simulink model "ELEC522_PROJECT2"  (Simulink 8.9)
settings: Solver=VariableStepAuto  StartTime=0.0  StopTime=10  RelTol=1e-3
undefined symbols (not defined in the file): A, N
libraries: xbsIndex_r4 x127, JTAGRuntimeCosim_r4 x1
(part 1 of 2)
settings Model: Creator=Kenny_LR  LastModifiedBy=rl59
settings DataIOCC: LimitDataPoints=off  SaveFormat=Dataset  SignalLoggingSaveFormat=Dataset
settings OptimizationCC: LifeSpan=auto
settings DebuggingCC: UnderspecifiedInitializationDetection=Simplified  MergeDetectMultiDrivingBlocksExec=error  FcnCallInpInsideContextMsg=error  StateNameClashWarn=none  SFUnexpectedBacktrackingDiag=error  SFNoUnconditionalDefaultTransitionDiag=error  SFExecutionAtInitializationDiag=warning
settings HardwareCC: ProdBitPerPointer=64  ProdBitPerSizeT=64  ProdBitPerPtrDiffT=64  ProdLargestAtomicFloat=Float  ProdIntDivRoundTo=Zero  ProdEndianess=LittleEndian  ProdWordSize=64  ProdHWDeviceType=Intel->x86-64 (Windows64)
settings ModelReferenceCC: PropagateSignalLabelsOutOfModel=on
settings GRTTargetCC: TargetLangStandard=C99 (ISO)  GeneratePreprocessorConditionals=Use local settings  CombineOutputUpdateFcns=on  GRTInterface=off
settings ConfigComp: CovMetricSettings=dwe  CovHtmlReporting=off  CovSaveCumulativeToWorkspaceVar=off  CovSaveSingleToWorkspaceVar=off  CovExternalEMLEnable=on

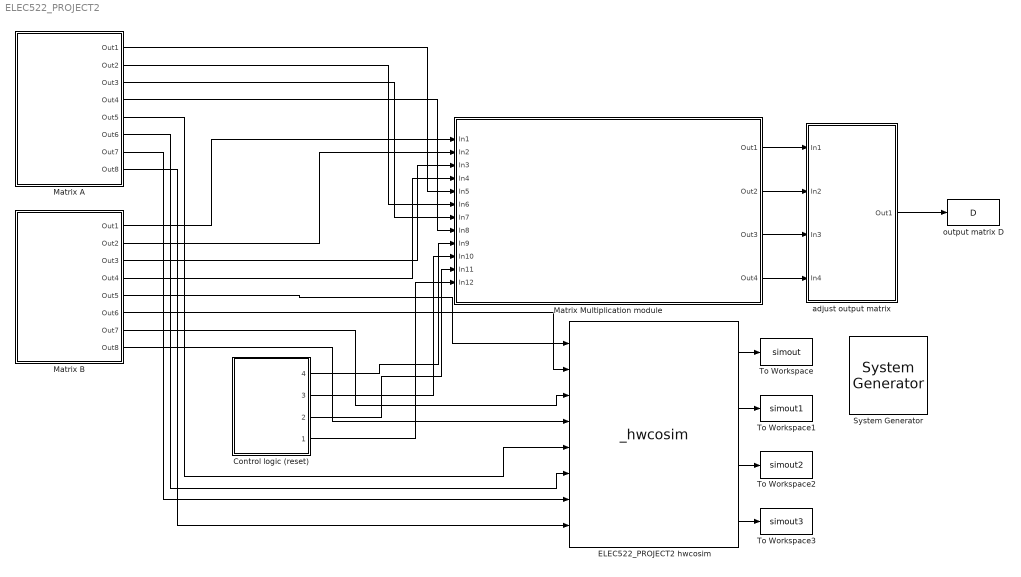
== system ELEC522_PROJECT2 ==
  " System Generator" : xbsIndex_r4/ System Generator  Tag=genX  xilinxfamily=zynq  part=xc7z020  speed=-1  package=clg484  synthesis_tool=Vivado  clock_wrapper=Clock Enables  directory=./netlist  proj_type=Vivado  Synth_file=Vivado Synthesis Defaults  Impl_file=Vivado Implementation Defaults  testbench=off  simulink_period=1  sysclk_period=10  dcm_input_clock_period=10  incr_netlist=off  trim_vbits=Everywhere in SubSystem  dbl_ovrd=According to Block Masks  core_generation=According to Block Masks  run_coregen=off  deprecated_control=off  eval_field=0  block_type=sysgen
  Control logic (reset) : Subsystem
  ELEC522_PROJECT2 hwcosim : JTAGRuntimeCosim_r4/_hwcosim  clkSrc=Single Stepped  hasCombinationalPath=on  bitfileName=C:\Users\rl59\Desktop\netlist\elec522_project2.bit  skipConfig=off  dispPartInfo=off  useZynqReconfigScript=on  cable=Auto Detect  speed=N/A  cablePort=N/A  cableLocation=Local  shareCable=off  design_xtable=|  engineDll=JTAGCosimEngine.dll  cableWaitTime=10  bscanPos=-1  IRLengths=[]  useWaitBox=1  hasBufgmux=on  Scheme=Cosim  useCmdProc=1  hasProc=0  useImpact=0  printLogFile=0  userChain=2  block_type=jtagcosim
      | {
      |     'clkWrapper' => 'elec522_project2',
      |     'burstMode' => false,
      |     'burstFifoDepth' => '1024',
      |     'shared_memories' => {},
      |     'clocksGcd' => 1,
      |     'device' => {
      |       'family' => 'zynq',
      |       'part' => 'xc7z020',
      |       'package' => 'clg484',
      |       'speed' => '-1',
      |     },
      |     'ports' => {
      |       'gateway_in3' => {
      |         'direction' => 'in',
      |         'width' => 16,
      |         'name' => 'gateway_in3',
      |         'period' => 1,
      |         'icon_text' => 'Gateway In3',
      |         'type' => 'UFix_16_0',
      |         'arithmetic_type' => 'xlUnsigned',
      |         'dat_file' => 'elec522_project2_matrix_b_gateway_in3.dat',
      |         'bin_pt' => 0,
      |         'addr_offset' => 0,
      |         'bd_port_index' => 0,
      |       },
      |       'gateway_in2' => {
      |         'direction' => 'in',
      |         'width' => 16,
      |         'name' => 'gateway_in2',
      |         'period' => 1,
      |         'icon_text' => 'Gateway In2',
      |         'type' => 'UFix_16_0',
      |         'arithmetic_type' => 'xlUnsigned',
      |         'dat_file' => 'elec522_project2_matrix_b_gateway_in2.dat',
      |         'bin_pt' => 0,
      |         'addr_offset' => 4,
      |         'bd_port_index' => 1,
      |       },
      |       'gateway_in1' => {
      |         'direction' => 'in',
      |         'width' => 16,
      |         'name' => 'gateway_in1',
      |         'period' => 1,
      |         'icon_text' => 'Gateway In1',
      |         'type' => 'UFix_16_0',
      |         'arithmetic_type' => 'xlUnsigned',
      |         'dat_file' => 'elec522_project2_matrix_b_gateway_in1.dat',
      |         'bin_pt' => 0,
      |         'addr_offset' => 8,
      |         'bd_port_index' => 2,
      |       },
      |       'gateway_in' => {
      |         'direction' => 'in',
      |         'width' => 16,
      |         'name' => 'gateway_in',
      |         'period' => 1,
      |         'icon_text' => 'Gateway In',
      |         'type' => 'UFix_16_0',
      |         'arithmetic_type' => 'xlUnsigned',
      |         'dat_file' => 'elec522_project2_matrix_b_gateway_in.dat',
      |         'bin_pt' => 0,
      |         'addr_offset' => 12,
      |         'bd_port_index' => 3,
      |       },
      |       'gateway_in7' => {
      |         'direction' => 'in',
      |         'width' => 16,
      |         'name' => 'gateway_in7',
      |         'period' => 1,
      |         'icon_text' => 'Gateway In7',
      |         'type' => 'UFix_16_0',
      |         'arithmetic_type' => 'xlUnsigned',
      |         'dat_file' => 'elec522_project2_matrix_a_gateway_in7.dat',
      |         'bin_pt' => 0,
      |         'addr_offset' => 16,
      |         'bd_port_index' => 4,
      |       },
      |       'gateway_in6' => {
      |         'direction' => 'in',
      |         'width' => 16,
      |         'name' => 'gateway_in6',
      |         'period' => 1,
      |         'icon_text' => 'Gateway In6',
      |         'type' => 'UFix_16_0',
      |         'arithmetic_type' => 'xlUnsigned',
      |         'dat_file' => 'elec522_project2_matrix_a_gateway_in6.dat',
      |         'bin_pt' => 0,
      |         'addr_offset' => 20,
      |         'bd_port_index' => 5,
      |       },
      |       'gateway_in5' => {
      |         'direction' => 'in',
      |         'width' => 16,
      |         'name' => 'gateway_in5',
      |         'period' => 1,
      |         'icon_text' => 'Gateway In5',
      |         'type' => 'UFix_16_0',
      |         'arithmetic_type' => 'xlUnsigned',
      |         'dat_file' => 'elec522_project2_matrix_a_gateway_in5.dat',
      |         'bin_pt' => 0,
      |         'addr_offset' => 24,
      |         'bd_port_index' => 6,
      |       },
      |       'gateway_in4' => {
      |         'direction' => 'in',
      |         'width' => 16,
      |         'name' => 'gateway_in4',
      |         'period' => 1,
      |         'icon_text' => 'Gateway In4',
      |         'type' => 'UFix_16_0',
      |         'arithmetic_type' => 'xlUnsigned',
      |         'dat_file' => 'elec522_project2_matrix_a_gateway_in4.dat',
      |         'bin_pt' => 0,
      |         'addr_offset' => 28,
      |         'bd_port_index' => 7,
      |       },
      |       'gateway_out' => {
      |         'direction' => 'out',
      |         'width' => 28,
      |         'name' => 'gateway_out',
      |         'period' => 1,
      |         'icon_text' => 'Gateway Out',
      |         'type' => 'UFix_28_0',
      |         'arithmetic_type' => 'xlUnsigned',
      |         'dat_file' => 'elec522_project2_adjust_output_matrix_gateway_out.dat',
      |         'bin_pt' => 0,
      |         'addr_offset' => 32,
      |         'bd_port_index' => 0,
      |       },
      |       'gateway_out1' => {
      |         'direction' => 'out',
      |         'width' => 28,
      |         'name' => 'gateway_out1',
      |         'period' => 1,
      |         'icon_text' => 'Gateway Out1',
      |         'type' => 'UFix_28_0',
      |         'arithmetic_type' => 'xlUnsigned',
      |         'dat_file' => 'elec522_project2_adjust_output_matrix_gateway_out1.dat',
      |         'bin_pt' => 0,
      |         'addr_offset' => 36,
      |         'bd_port_index' => 1,
      |       },
      |       'gateway_out2' => {
      |         'direction' => 'out',
      |         'width' => 28,
      |         'name' => 'gateway_out2',
      |         'period' => 1,
      |         'icon_text' => 'Gateway Out2',
      |         'type' => 'UFix_28_0',
      |         'arithmetic_type' => 'xlUnsigned',
      |         'dat_file' => 'elec522_project2_adjust_output_matrix_gateway_out2.dat',
      |         'bin_pt' => 0,
      |         'addr_offset' => 40,
      |         'bd_port_index' => 2,
      |       },
      |       'gateway_out3' => {
      |         'direction' => 'out',
      |         'width' => 28,
      |         'name' => 'gateway_out3',
      |         'period' => 1,
      |         'icon_text' => 'Gateway Out3',
      |         'type' => 'UFix_28_0',
      |         'arithmetic_type' => 'xlUnsigned',
      |         'dat_file' => 'elec522_project2_adjust_output_matrix_gateway_out3.dat',
      |         'bin_pt' => 0,
      |         'addr_offset' => 44,
      |         'bd_port_index' => 3,
      |       },
      |     },
      |   }
  Matrix A : Subsystem
  Matrix B : Subsystem
  Matrix Multiplication module : Subsystem
  To Workspace : ToWorkspace  VariableName=simout  SaveFormat=Timeseries  SampleTime=-1
  To Workspace1 : ToWorkspace  VariableName=simout1  SaveFormat=Timeseries  SampleTime=-1
  To Workspace2 : ToWorkspace  VariableName=simout2  SaveFormat=Timeseries  SampleTime=-1
  To Workspace3 : ToWorkspace  VariableName=simout3  SaveFormat=Timeseries  SampleTime=-1
  "adjust output matrix " : Subsystem
  output matrix D : ToWorkspace  VariableName=D  SampleTime=1
      settings: MaxDataPoints=4
  wires:
  Control logic (reset)/1(4) -> Matrix Multiplication module/9(In9)
  Control logic (reset)/2(3) -> Matrix Multiplication module/10(In10)
  Control logic (reset)/3(2) -> Matrix Multiplication module/11(In11)
  Control logic (reset)/4(1) -> Matrix Multiplication module/12(In12)
  ELEC522_PROJECT2 hwcosim/1 -> To Workspace/1
  ELEC522_PROJECT2 hwcosim/2 -> To Workspace1/1
  ELEC522_PROJECT2 hwcosim/3 -> To Workspace2/1
  ELEC522_PROJECT2 hwcosim/4 -> To Workspace3/1
  Matrix A/1(Out1) -> Matrix Multiplication module/5(In5)
  Matrix A/2(Out2) -> Matrix Multiplication module/6(In6)
  Matrix A/3(Out3) -> Matrix Multiplication module/7(In7)
  Matrix A/4(Out4) -> Matrix Multiplication module/8(In8)
  Matrix A/5(Out5) -> ELEC522_PROJECT2 hwcosim/5
  Matrix A/6(Out6) -> ELEC522_PROJECT2 hwcosim/6
  Matrix A/7(Out7) -> ELEC522_PROJECT2 hwcosim/7
  Matrix A/8(Out8) -> ELEC522_PROJECT2 hwcosim/8
  Matrix B/1(Out1) -> Matrix Multiplication module/1(In1)
  Matrix B/2(Out2) -> Matrix Multiplication module/2(In2)
  Matrix B/3(Out3) -> Matrix Multiplication module/3(In3)
  Matrix B/4(Out4) -> Matrix Multiplication module/4(In4)
  Matrix B/5(Out5) -> ELEC522_PROJECT2 hwcosim/1
  Matrix B/6(Out6) -> ELEC522_PROJECT2 hwcosim/2
  Matrix B/7(Out7) -> ELEC522_PROJECT2 hwcosim/3
  Matrix B/8(Out8) -> ELEC522_PROJECT2 hwcosim/4
  Matrix Multiplication module/1(Out1) -> "adjust output matrix "/1(In1)
  Matrix Multiplication module/2(Out2) -> "adjust output matrix "/2(In2)
  Matrix Multiplication module/3(Out3) -> "adjust output matrix "/3(In3)
  Matrix Multiplication module/4(Out4) -> "adjust output matrix "/4(In4)
  "adjust output matrix "/1(Out1) -> output matrix D/1

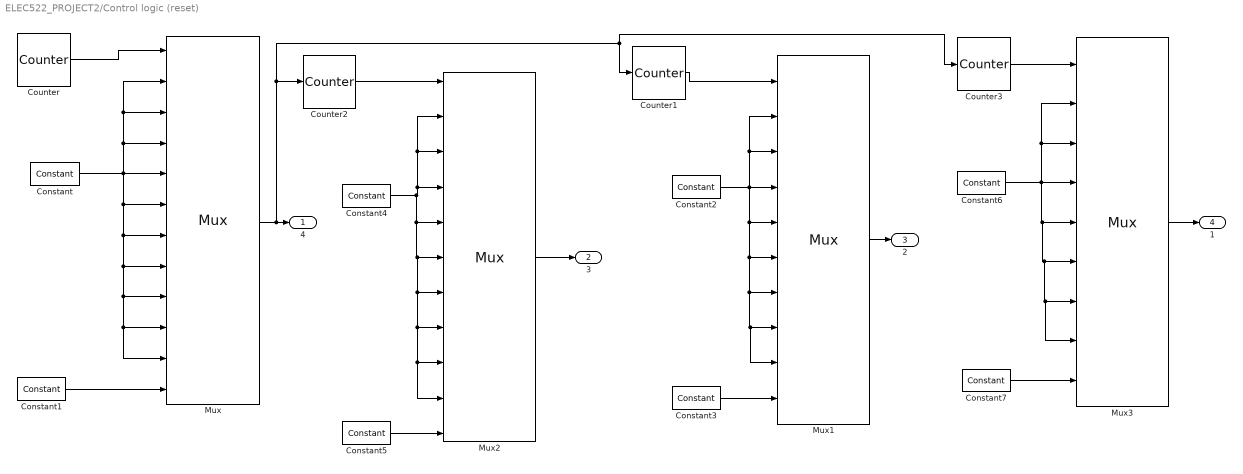
== system ELEC522_PROJECT2/Control logic (reset) ==
  Constant{,2,4,6} (4 alike) : xbsIndex_r4/Constant  const=0  gui_display_data_type=Boolean  arith_type=Boolean  n_bits=1  bin_pt=0  preci_type=Single  exp_width=8  frac_width=24  explicit_period=on  period=1  equ=P=C  opselect=C  inp2=PCIN>>17  opr=+  inp1=P  carry=CIN  dbl_ovrd=off  block_type=constant
  Constant{1,3,5,7} (4 alike) : xbsIndex_r4/Constant  const=1  gui_display_data_type=Boolean  arith_type=Boolean  n_bits=1  bin_pt=0  preci_type=Single  exp_width=8  frac_width=24  explicit_period=on  period=1  equ=P=C  opselect=C  inp2=PCIN>>17  opr=+  inp1=P  carry=CIN  dbl_ovrd=off  block_type=constant
  Counter : xbsIndex_r4/Counter  cnt_type=Count Limited  cnt_to=10  operation=Up  start_count=0  cnt_by_val=1  arith_type=Unsigned  n_bits=4  bin_pt=0  load_pin=off  rst=off  en=off  explicit_period=on  period=1  use_behavioral_HDL=off  implementation=Fabric  dbl_ovrd=off  block_type=counter
  Counter1 : xbsIndex_r4/Counter  cnt_type=Count Limited  cnt_to=8  operation=Up  start_count=0  cnt_by_val=1  arith_type=Unsigned  n_bits=4  bin_pt=0  load_pin=off  rst=on  en=off  explicit_period=on  period=1  use_behavioral_HDL=off  implementation=Fabric  dbl_ovrd=off  block_type=counter
  Counter2 : xbsIndex_r4/Counter  cnt_type=Count Limited  cnt_to=9  operation=Up  start_count=0  cnt_by_val=1  arith_type=Unsigned  n_bits=4  bin_pt=0  load_pin=off  rst=on  en=off  explicit_period=on  period=1  use_behavioral_HDL=off  implementation=Fabric  dbl_ovrd=off  block_type=counter
  Counter3 : xbsIndex_r4/Counter  cnt_type=Count Limited  cnt_to=7  operation=Up  start_count=0  cnt_by_val=1  arith_type=Unsigned  n_bits=3  bin_pt=0  load_pin=off  rst=on  en=off  explicit_period=on  period=1  use_behavioral_HDL=off  implementation=Fabric  dbl_ovrd=off  block_type=counter
  Mux : xbsIndex_r4/Mux  inputs=11  en=off  latency=0  precision=Full  arith_type=Unsigned  n_bits=16  bin_pt=14  quantization=Truncate  overflow=Wrap  dbl_ovrd=off  block_type=mux
  Mux1 : xbsIndex_r4/Mux  inputs=9  en=off  latency=0  precision=Full  arith_type=Unsigned  n_bits=16  bin_pt=14  quantization=Truncate  overflow=Wrap  dbl_ovrd=off  block_type=mux
  Mux2 : xbsIndex_r4/Mux  inputs=10  en=off  latency=0  precision=Full  arith_type=Unsigned  n_bits=16  bin_pt=14  quantization=Truncate  overflow=Wrap  dbl_ovrd=off  block_type=mux
  Mux3 : xbsIndex_r4/Mux  inputs=8  en=off  latency=0  precision=Full  arith_type=Unsigned  n_bits=16  bin_pt=14  quantization=Truncate  overflow=Wrap  dbl_ovrd=off  block_type=mux
  4 : Outport
  3 : Outport  Port=2
  2 : Outport  Port=3
  1 : Outport  Port=4
  wires:
  Mux/1 -> Counter3/1, Counter1/1, Counter2/1, 4/1
  Counter/1 -> Mux/1
  Constant1/1 -> Mux/12
  Counter1/1 -> Mux1/1
  Counter2/1 -> Mux2/1
  Counter3/1 -> Mux3/1
  Constant5/1 -> Mux2/11
  Constant3/1 -> Mux1/10
  Mux2/1 -> 3/1
  Mux1/1 -> 2/1
  Mux3/1 -> 1/1
  Constant7/1 -> Mux3/9
  Constant/1 -> Mux/11, Mux/10, Mux/9, Mux/8, Mux/7, Mux/6, Mux/5, Mux/4, Mux/3, Mux/2
  Constant4/1 -> Mux2/10, Mux2/9, Mux2/8, Mux2/7, Mux2/6, Mux2/5, Mux2/4, Mux2/3, Mux2/2
  Constant2/1 -> Mux1/9, Mux1/8, Mux1/7, Mux1/6, Mux1/5, Mux1/4, Mux1/3, Mux1/2
  Constant6/1 -> Mux3/8, Mux3/7, Mux3/6, Mux3/5, Mux3/4, Mux3/3, Mux3/2

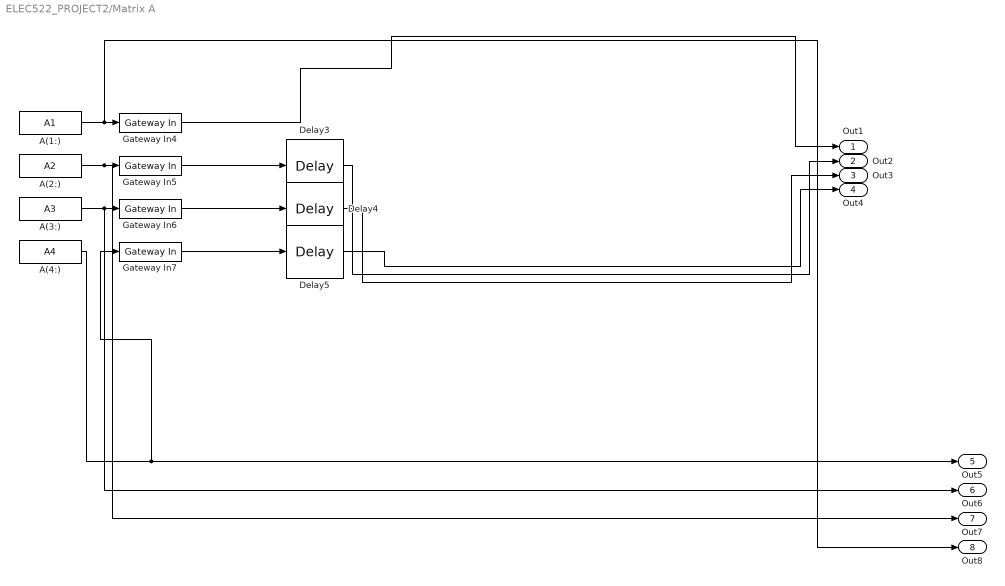
== system ELEC522_PROJECT2/Matrix A ==
  A(1:) : FromWorkspace  VariableName=A1  SampleTime=1  OutputAfterFinalValue=Setting to zero
  A(2:) : FromWorkspace  VariableName=A2  SampleTime=0  OutputAfterFinalValue=Setting to zero
  A(3:) : FromWorkspace  VariableName=A3  SampleTime=0  OutputAfterFinalValue=Setting to zero
  A(4:) : FromWorkspace  VariableName=A4  SampleTime=0  OutputAfterFinalValue=Setting to zero
  Delay3 : xbsIndex_r4/Delay  rst=off  infoeditControl=Selection of Reset will increase slice count due to use of real FFs and instead of SRLs  en=off  latency=1  reg_retiming=off  dbl_ovrd=off  block_type=delay
  Delay4 : xbsIndex_r4/Delay  rst=off  infoeditControl=Selection of Reset will increase slice count due to use of real FFs and instead of SRLs  en=off  latency=2  reg_retiming=off  dbl_ovrd=off  block_type=delay
  Delay5 : xbsIndex_r4/Delay  rst=off  infoeditControl=Selection of Reset will increase slice count due to use of real FFs and instead of SRLs  en=off  latency=3  reg_retiming=off  dbl_ovrd=off  block_type=delay
  Gateway In{4..7} (4 alike) : xbsIndex_r4/Gateway In  gui_display_data_type=Fixed-point  arith_type=Unsigned  n_bits=16  bin_pt=0  preci_type=Single  exp_width=8  frac_width=24  rows=1  columns=1  quantization="Round  (unbiased: +/- Inf)"  overflow=Saturate  period=1  UseAsADC=off  ADCChannel='1'  interface=None  automatic_assignment=on  address_offset=hex2dec('00')  intf_name=''  intf_description=''  default_value=0  timing_constraint=None  locs_specified=off  LOCs={}  io_standard={}  inherit_from_input=off  hdl_port=on  dbl_ovrd=off  block_type=gatewayin
  Out1 : Outport
  Out2 : Outport  Port=2
  Out3 : Outport  Port=3
  Out4 : Outport  Port=4
  Out5 : Outport  Port=5
  Out6 : Outport  Port=6
  Out7 : Outport  Port=7
  Out8 : Outport  Port=8
  wires:
  Gateway In6/1 -> Delay4/1
  A(2:)/1 -> Out7/1, Gateway In5/1
  Gateway In5/1 -> Delay3/1
  Gateway In7/1 -> Delay5/1
  A(1:)/1 -> Out8/1, Gateway In4/1
  A(3:)/1 -> Out6/1, Gateway In6/1
  A(4:)/1 -> Out5/1, Gateway In7/1
  Gateway In4/1 -> Out1/1
  Delay3/1 -> Out2/1
  Delay4/1 -> Out3/1
  Delay5/1 -> Out4/1

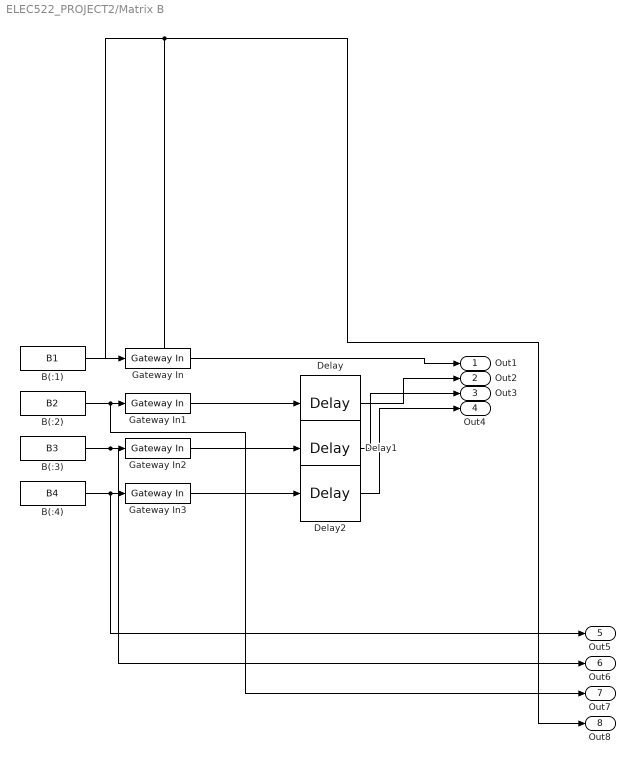
== system ELEC522_PROJECT2/Matrix B ==
  B(:1) : FromWorkspace  VariableName=B1  SampleTime=1  OutputAfterFinalValue=Setting to zero
  B(:2) : FromWorkspace  VariableName=B2  SampleTime=1  OutputAfterFinalValue=Setting to zero
  B(:3) : FromWorkspace  VariableName=B3  SampleTime=1  OutputAfterFinalValue=Setting to zero
  B(:4) : FromWorkspace  VariableName=B4  SampleTime=1  OutputAfterFinalValue=Setting to zero
  Delay : xbsIndex_r4/Delay  rst=off  infoeditControl=Selection of Reset will increase slice count due to use of real FFs and instead of SRLs  en=off  latency=1  reg_retiming=off  dbl_ovrd=off  block_type=delay
  Delay1 : xbsIndex_r4/Delay  rst=off  infoeditControl=Selection of Reset will increase slice count due to use of real FFs and instead of SRLs  en=off  latency=2  reg_retiming=off  dbl_ovrd=off  block_type=delay
  Delay2 : xbsIndex_r4/Delay  rst=off  infoeditControl=Selection of Reset will increase slice count due to use of real FFs and instead of SRLs  en=off  latency=3  reg_retiming=off  dbl_ovrd=off  block_type=delay
  Gateway In{,1..3} (4 alike) : xbsIndex_r4/Gateway In  gui_display_data_type=Fixed-point  arith_type=Unsigned  n_bits=16  bin_pt=0  preci_type=Single  exp_width=8  frac_width=24  rows=1  columns=1  quantization="Round  (unbiased: +/- Inf)"  overflow=Saturate  period=1  UseAsADC=off  ADCChannel='1'  interface=None  automatic_assignment=on  address_offset=hex2dec('00')  intf_name=''  intf_description=''  default_value=0  timing_constraint=None  locs_specified=off  LOCs={}  io_standard={}  inherit_from_input=off  hdl_port=on  dbl_ovrd=off  block_type=gatewayin
  Out1 : Outport
  Out2 : Outport  Port=2
  Out3 : Outport  Port=3
  Out4 : Outport  Port=4
  Out5 : Outport  Port=5
  Out6 : Outport  Port=6
  Out7 : Outport  Port=7
  Out8 : Outport  Port=8
  wires:
  B(:2)/1 -> Out7/1, Gateway In1/1
  B(:1)/1 -> Out8/1, Gateway In/1
  B(:3)/1 -> Out6/1, Gateway In2/1
  Gateway In2/1 -> Delay1/1
  Gateway In3/1 -> Delay2/1
  Gateway In1/1 -> Delay/1
  B(:4)/1 -> Out5/1, Gateway In3/1
  Gateway In/1 -> Out1/1
  Delay/1 -> Out2/1
  Delay1/1 -> Out3/1
  Delay2/1 -> Out4/1

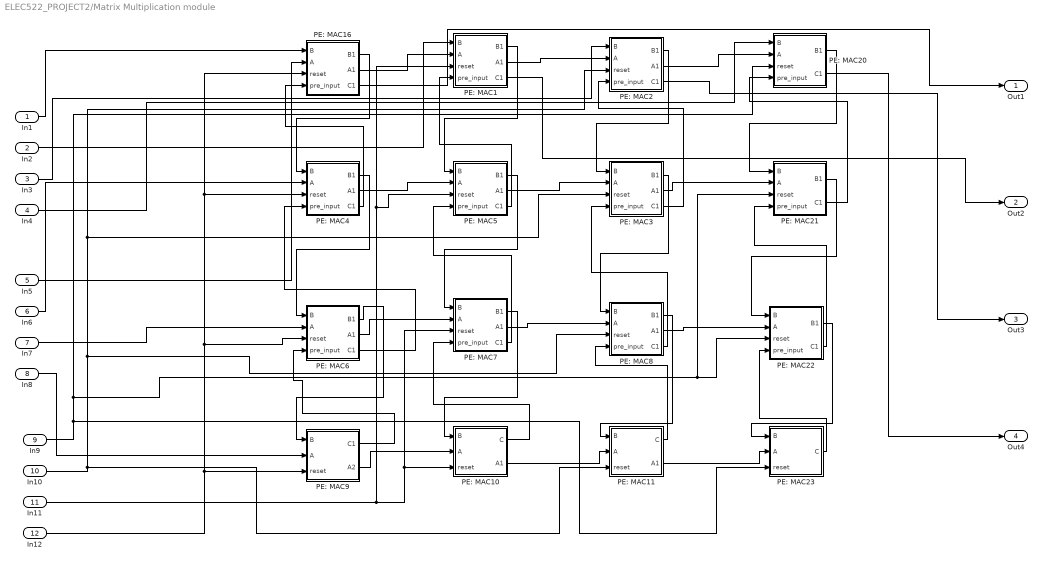
== system ELEC522_PROJECT2/Matrix Multiplication module ==
  In1 : Inport
  In2 : Inport  Port=2
  In3 : Inport  Port=3
  In4 : Inport  Port=4
  In5 : Inport  Port=5
  In6 : Inport  Port=6
  In7 : Inport  Port=7
  In8 : Inport  Port=8
  In9 : Inport  Port=9
  In10 : Inport  Port=10
  In11 : Inport  Port=11
  In12 : Inport  Port=12
  PE: MAC1 : Subsystem
  PE: MAC10 : Subsystem
  PE: MAC11 : Subsystem
  PE: MAC16 : Subsystem
  PE: MAC2 : Subsystem
  PE: MAC20 : Subsystem
  PE: MAC21 : Subsystem
  PE: MAC22 : Subsystem
  PE: MAC23 : Subsystem
  PE: MAC3 : Subsystem
  PE: MAC4 : Subsystem
  PE: MAC5 : Subsystem
  PE: MAC6 : Subsystem
  PE: MAC7 : Subsystem
  PE: MAC8 : Subsystem
  PE: MAC9 : Subsystem
  Out1 : Outport
  Out2 : Outport  Port=2
  Out3 : Outport  Port=3
  Out4 : Outport  Port=4
  wires:
  PE: MAC10/1(C) -> PE: MAC7/4(pre_input)
  PE: MAC11/2(A1) -> PE: MAC23/2(A)
  PE: MAC7/3(C1) -> PE: MAC5/4(pre_input)
  PE: MAC5/3(C1) -> PE: MAC1/4(pre_input)
  PE: MAC2/1(B1) -> PE: MAC3/1(B)
  In7/1 -> PE: MAC6/2(A)
  In2/1 -> PE: MAC1/1(B)
  PE: MAC22/1(B1) -> PE: MAC23/1(B)
  PE: MAC6/2(A1) -> PE: MAC7/2(A)
  PE: MAC4/3(C1) -> PE: MAC16/4(pre_input)
  In4/1 -> PE: MAC20/1(B)
  PE: MAC8/1(B1) -> PE: MAC11/1(B)
  PE: MAC6/3(C1) -> PE: MAC4/4(pre_input)
  PE: MAC11/1(C) -> PE: MAC8/4(pre_input)
  PE: MAC21/2(C1) -> PE: MAC20/4(pre_input)
  In5/1 -> PE: MAC16/2(A)
  PE: MAC20/1(B1) -> PE: MAC21/1(B)
  PE: MAC16/1(B1) -> PE: MAC4/1(B)
  In1/1 -> PE: MAC16/1(B)
  PE: MAC7/2(A1) -> PE: MAC8/2(A)
  PE: MAC7/1(B1) -> PE: MAC10/1(B)
  PE: MAC3/3(C1) -> PE: MAC2/4(pre_input)
  In6/1 -> PE: MAC4/2(A)
  PE: MAC8/2(A1) -> PE: MAC22/2(A)
  PE: MAC2/2(A1) -> PE: MAC20/2(A)
  PE: MAC21/1(B1) -> PE: MAC22/1(B)
  PE: MAC9/1(C1) -> PE: MAC6/4(pre_input)
  PE: MAC6/1(B1) -> PE: MAC9/1(B)
  PE: MAC4/1(B1) -> PE: MAC6/1(B)
  In8/1 -> PE: MAC9/2(A)
  PE: MAC5/2(A1) -> PE: MAC3/2(A)
  In3/1 -> PE: MAC2/1(B)
  PE: MAC1/1(B1) -> PE: MAC5/1(B)
  PE: MAC4/2(A1) -> PE: MAC5/2(A)
  PE: MAC1/2(A1) -> PE: MAC2/2(A)
  PE: MAC8/3(C1) -> PE: MAC3/4(pre_input)
  PE: MAC16/2(A1) -> PE: MAC1/2(A)
  PE: MAC5/1(B1) -> PE: MAC7/1(B)
  PE: MAC3/1(B1) -> PE: MAC8/1(B)
  PE: MAC23/1(C) -> PE: MAC22/4(pre_input)
  PE: MAC22/2(C1) -> PE: MAC21/4(pre_input)
  PE: MAC3/2(A1) -> PE: MAC21/2(A)
  PE: MAC9/2(A2) -> PE: MAC10/2(A)
  PE: MAC10/2(A1) -> PE: MAC11/2(A)
  In11/1 -> PE: MAC10/3(reset), PE: MAC7/3(reset), PE: MAC5/3(reset), PE: MAC1/3(reset)
  In10/1 -> PE: MAC11/3(reset), PE: MAC8/3(reset), PE: MAC3/3(reset), PE: MAC2/3(reset)
  In12/1 -> PE: MAC9/3(reset), PE: MAC6/3(reset), PE: MAC4/3(reset), PE: MAC16/3(reset)
  In9/1 -> PE: MAC23/3(reset), PE: MAC21/3(reset), PE: MAC22/3(reset), PE: MAC20/3(reset)
  PE: MAC20/2(C1) -> Out4/1
  PE: MAC2/3(C1) -> Out3/1
  PE: MAC16/3(C1) -> Out1/1
  PE: MAC1/3(C1) -> Out2/1

== system ELEC522_PROJECT2/adjust output matrix  ==
  In1 : Inport
  In2 : Inport  Port=2
  In3 : Inport  Port=3
  In4 : Inport  Port=4
  Gateway Out{,1..3} (4 alike) : xbsIndex_r4/Gateway Out  inherit_from_input=off  hdl_port=on  rows=1  columns=1  UseAsDAC=off  DACChannel='1'  interface=None  automatic_assignment=on  address_offset=hex2dec('00')  intf_name=''  intf_description=''  timing_constraint=None  locs_specified=off  LOCs={}  io_standard={}  block_type=gatewayout
  MATLAB Function1 : MATLAB Function  TreatAsAtomicUnit=on
  Out1 : Outport
  wires:
  In2/1 -> Gateway Out1/1
  In1/1 -> Gateway Out/1
  In4/1 -> Gateway Out3/1
  In3/1 -> Gateway Out2/1
  Gateway Out3/1 -> MATLAB Function1/4(c4)
  Gateway Out2/1 -> MATLAB Function1/3(c3)
  Gateway Out/1 -> MATLAB Function1/1(c1)
  Gateway Out1/1 -> MATLAB Function1/2(c2)
  MATLAB Function1/1(y) -> Out1/1

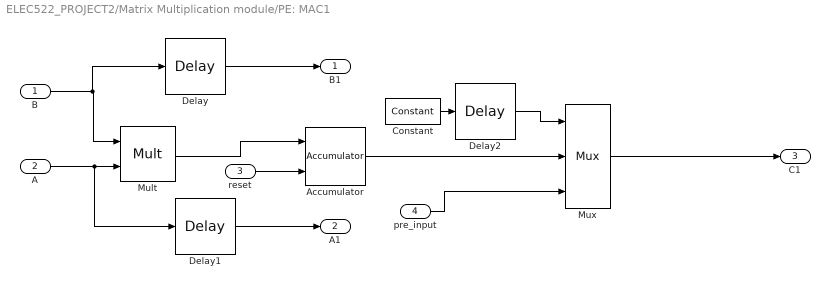
== system ELEC522_PROJECT2/Matrix Multiplication module/PE: MAC1 ==
  B : Inport
  A : Inport  Port=2
  reset : Inport  Port=3
  pre_input : Inport  Port=4
  Accumulator : xbsIndex_r4/Accumulator  operation=Add  n_bits=28  overflow=Wrap  scale=1  rst=on  hasbypass=off  infoeditControl=reset for floating point data type must be asserted for a minimum of 2 cycles  en=off  latency=1  msb_inp=100  msb=100  lsb=-100  use_behavioral_HDL=on  implementation=Fabric  dbl_ovrd=off  block_type=accum
  Constant : xbsIndex_r4/Constant  const=1.0  gui_display_data_type=Boolean  arith_type=Boolean  n_bits=16  bin_pt=14  preci_type=Single  exp_width=8  frac_width=24  explicit_period=on  period=1  equ=P=C  opselect=C  inp2=PCIN>>17  opr=+  inp1=P  carry=CIN  dbl_ovrd=off  block_type=constant
  Delay : xbsIndex_r4/Delay  rst=off  infoeditControl=Selection of Reset will increase slice count due to use of real FFs and instead of SRLs  en=off  latency=1  reg_retiming=off  dbl_ovrd=off  block_type=delay
  Delay1 : xbsIndex_r4/Delay  rst=off  infoeditControl=Selection of Reset will increase slice count due to use of real FFs and instead of SRLs  en=off  latency=1  reg_retiming=off  dbl_ovrd=off  block_type=delay
  Delay2 : xbsIndex_r4/Delay  rst=off  infoeditControl=Selection of Reset will increase slice count due to use of real FFs and instead of SRLs  en=off  latency=6  reg_retiming=off  dbl_ovrd=off  block_type=delay
  Mult : xbsIndex_r4/Mult  precision=Full  arith_type="Signed  (2's comp)"  n_bits=16  bin_pt=14  quantization=Truncate  overflow=Wrap  en=off  latency=0  use_behavioral_HDL=off  opt=Speed  use_embedded=on  optimum_pipeline=off  pipeline=on  dbl_ovrd=off  use_rpm=on  placement_style=Triangular  block_type=mult
  Mux : xbsIndex_r4/Mux  inputs=2  en=off  latency=2  precision=Full  arith_type=Unsigned  n_bits=16  bin_pt=14  quantization=Truncate  overflow=Wrap  dbl_ovrd=off  block_type=mux
  B1 : Outport
  A1 : Outport  Port=2
  C1 : Outport  Port=3
  wires:
  A/1 -> Delay1/1, Mult/2
  B/1 -> Delay/1, Mult/1
  Mult/1 -> Accumulator/1
  Delay1/1 -> A1/1
  Delay/1 -> B1/1
  reset/1 -> Accumulator/2
  Accumulator/1 -> Mux/2
  Constant/1 -> Delay2/1
  Delay2/1 -> Mux/1
  pre_input/1 -> Mux/3
  Mux/1 -> C1/1

== system ELEC522_PROJECT2/Matrix Multiplication module/PE: MAC10 ==
  B : Inport
  A : Inport  Port=2
  reset : Inport  Port=3
  Accumulator : xbsIndex_r4/Accumulator  operation=Add  n_bits=28  overflow=Wrap  scale=1  rst=on  hasbypass=off  infoeditControl=reset for floating point data type must be asserted for a minimum of 2 cycles  en=off  latency=1  msb_inp=100  msb=100  lsb=-100  use_behavioral_HDL=on  implementation=Fabric  dbl_ovrd=off  block_type=accum
  Delay1 : xbsIndex_r4/Delay  rst=off  infoeditControl=Selection of Reset will increase slice count due to use of real FFs and instead of SRLs  en=off  latency=1  reg_retiming=off  dbl_ovrd=off  block_type=delay
  Mult : xbsIndex_r4/Mult  precision=Full  arith_type="Signed  (2's comp)"  n_bits=16  bin_pt=14  quantization=Truncate  overflow=Wrap  en=off  latency=0  use_behavioral_HDL=off  opt=Speed  use_embedded=on  optimum_pipeline=off  pipeline=on  dbl_ovrd=off  use_rpm=on  placement_style=Triangular  block_type=mult
  C : Outport
  A1 : Outport  Port=2
  wires:
  A/1 -> Delay1/1, Mult/2
  B/1 -> Mult/1
  Mult/1 -> Accumulator/1
  Delay1/1 -> A1/1
  reset/1 -> Accumulator/2
  Accumulator/1 -> C/1

== system ELEC522_PROJECT2/Matrix Multiplication module/PE: MAC11 ==
  B : Inport
  A : Inport  Port=2
  reset : Inport  Port=3
  Accumulator : xbsIndex_r4/Accumulator  operation=Add  n_bits=28  overflow=Wrap  scale=1  rst=on  hasbypass=off  infoeditControl=reset for floating point data type must be asserted for a minimum of 2 cycles  en=off  latency=1  msb_inp=100  msb=100  lsb=-100  use_behavioral_HDL=on  implementation=Fabric  dbl_ovrd=off  block_type=accum
  Delay1 : xbsIndex_r4/Delay  rst=off  infoeditControl=Selection of Reset will increase slice count due to use of real FFs and instead of SRLs  en=off  latency=1  reg_retiming=off  dbl_ovrd=off  block_type=delay
  Mult : xbsIndex_r4/Mult  precision=Full  arith_type="Signed  (2's comp)"  n_bits=16  bin_pt=14  quantization=Truncate  overflow=Wrap  en=off  latency=0  use_behavioral_HDL=off  opt=Speed  use_embedded=on  optimum_pipeline=off  pipeline=on  dbl_ovrd=off  use_rpm=on  placement_style=Triangular  block_type=mult
  C : Outport
  A1 : Outport  Port=2
  wires:
  A/1 -> Delay1/1, Mult/2
  B/1 -> Mult/1
  Mult/1 -> Accumulator/1
  Delay1/1 -> A1/1
  reset/1 -> Accumulator/2
  Accumulator/1 -> C/1

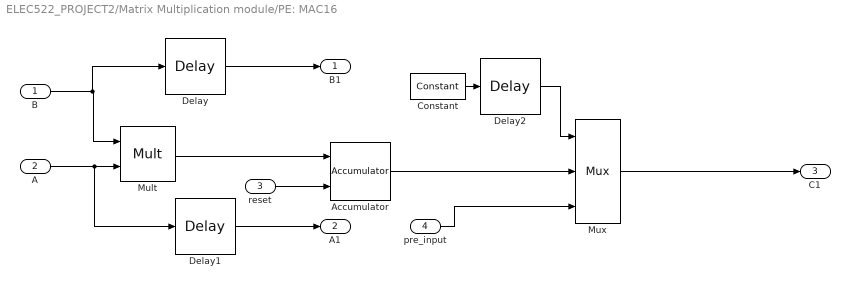
== system ELEC522_PROJECT2/Matrix Multiplication module/PE: MAC16 ==
  B : Inport
  A : Inport  Port=2
  reset : Inport  Port=3
  pre_input : Inport  Port=4
  Accumulator : xbsIndex_r4/Accumulator  operation=Add  n_bits=28  overflow=Wrap  scale=1  rst=on  hasbypass=off  infoeditControl=reset for floating point data type must be asserted for a minimum of 2 cycles  en=off  latency=1  msb_inp=100  msb=100  lsb=-100  use_behavioral_HDL=on  implementation=Fabric  dbl_ovrd=off  block_type=accum
  Constant : xbsIndex_r4/Constant  const=1.0  gui_display_data_type=Boolean  arith_type=Boolean  n_bits=16  bin_pt=14  preci_type=Single  exp_width=8  frac_width=24  explicit_period=on  period=1  equ=P=C  opselect=C  inp2=PCIN>>17  opr=+  inp1=P  carry=CIN  dbl_ovrd=off  block_type=constant
  Delay : xbsIndex_r4/Delay  rst=off  infoeditControl=Selection of Reset will increase slice count due to use of real FFs and instead of SRLs  en=off  latency=1  reg_retiming=off  dbl_ovrd=off  block_type=delay
  Delay1 : xbsIndex_r4/Delay  rst=off  infoeditControl=Selection of Reset will increase slice count due to use of real FFs and instead of SRLs  en=off  latency=1  reg_retiming=off  dbl_ovrd=off  block_type=delay
  Delay2 : xbsIndex_r4/Delay  rst=off  infoeditControl=Selection of Reset will increase slice count due to use of real FFs and instead of SRLs  en=off  latency=5  reg_retiming=off  dbl_ovrd=off  block_type=delay
  Mult : xbsIndex_r4/Mult  precision=Full  arith_type="Signed  (2's comp)"  n_bits=16  bin_pt=14  quantization=Truncate  overflow=Wrap  en=off  latency=0  use_behavioral_HDL=off  opt=Speed  use_embedded=on  optimum_pipeline=off  pipeline=on  dbl_ovrd=off  use_rpm=on  placement_style=Triangular  block_type=mult
  Mux : xbsIndex_r4/Mux  inputs=2  en=off  latency=3  precision=Full  arith_type=Unsigned  n_bits=16  bin_pt=14  quantization=Truncate  overflow=Wrap  dbl_ovrd=off  block_type=mux
  B1 : Outport
  A1 : Outport  Port=2
  C1 : Outport  Port=3
  wires:
  A/1 -> Delay1/1, Mult/2
  B/1 -> Delay/1, Mult/1
  Mult/1 -> Accumulator/1
  Delay1/1 -> A1/1
  Delay/1 -> B1/1
  reset/1 -> Accumulator/2
  Accumulator/1 -> Mux/2
  Constant/1 -> Delay2/1
  Delay2/1 -> Mux/1
  pre_input/1 -> Mux/3
  Mux/1 -> C1/1

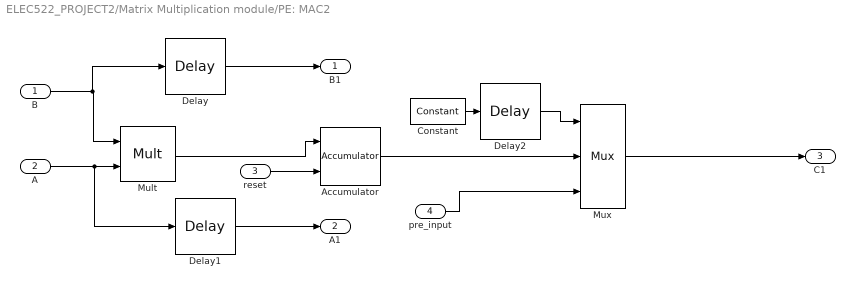
== system ELEC522_PROJECT2/Matrix Multiplication module/PE: MAC2 ==
  B : Inport
  A : Inport  Port=2
  reset : Inport  Port=3
  pre_input : Inport  Port=4
  Accumulator : xbsIndex_r4/Accumulator  operation=Add  n_bits=28  overflow=Wrap  scale=1  rst=on  hasbypass=off  infoeditControl=reset for floating point data type must be asserted for a minimum of 2 cycles  en=off  latency=1  msb_inp=100  msb=100  lsb=-100  use_behavioral_HDL=on  implementation=Fabric  dbl_ovrd=off  block_type=accum
  Constant : xbsIndex_r4/Constant  const=1.0  gui_display_data_type=Boolean  arith_type=Boolean  n_bits=16  bin_pt=14  preci_type=Single  exp_width=8  frac_width=24  explicit_period=on  period=1  equ=P=C  opselect=C  inp2=PCIN>>17  opr=+  inp1=P  carry=CIN  dbl_ovrd=off  block_type=constant
  Delay : xbsIndex_r4/Delay  rst=off  infoeditControl=Selection of Reset will increase slice count due to use of real FFs and instead of SRLs  en=off  latency=1  reg_retiming=off  dbl_ovrd=off  block_type=delay
  Delay1 : xbsIndex_r4/Delay  rst=off  infoeditControl=Selection of Reset will increase slice count due to use of real FFs and instead of SRLs  en=off  latency=1  reg_retiming=off  dbl_ovrd=off  block_type=delay
  Delay2 : xbsIndex_r4/Delay  rst=off  infoeditControl=Selection of Reset will increase slice count due to use of real FFs and instead of SRLs  en=off  latency=7  reg_retiming=off  dbl_ovrd=off  block_type=delay
  Mult : xbsIndex_r4/Mult  precision=Full  arith_type="Signed  (2's comp)"  n_bits=16  bin_pt=14  quantization=Truncate  overflow=Wrap  en=off  latency=0  use_behavioral_HDL=off  opt=Speed  use_embedded=on  optimum_pipeline=off  pipeline=on  dbl_ovrd=off  use_rpm=on  placement_style=Triangular  block_type=mult
  Mux : xbsIndex_r4/Mux  inputs=2  en=off  latency=1  precision=Full  arith_type=Unsigned  n_bits=16  bin_pt=14  quantization=Truncate  overflow=Wrap  dbl_ovrd=off  block_type=mux
  B1 : Outport
  A1 : Outport  Port=2
  C1 : Outport  Port=3
  wires:
  A/1 -> Delay1/1, Mult/2
  B/1 -> Delay/1, Mult/1
  Mult/1 -> Accumulator/1
  Delay1/1 -> A1/1
  Delay/1 -> B1/1
  reset/1 -> Accumulator/2
  Accumulator/1 -> Mux/2
  Constant/1 -> Delay2/1
  Delay2/1 -> Mux/1
  pre_input/1 -> Mux/3
  Mux/1 -> C1/1

== system ELEC522_PROJECT2/Matrix Multiplication module/PE: MAC20 ==
  B : Inport
  A : Inport  Port=2
  reset : Inport  Port=3
  pre_input : Inport  Port=4
  Accumulator : xbsIndex_r4/Accumulator  operation=Add  n_bits=28  overflow=Wrap  scale=1  rst=on  hasbypass=off  infoeditControl=reset for floating point data type must be asserted for a minimum of 2 cycles  en=off  latency=1  msb_inp=100  msb=100  lsb=-100  use_behavioral_HDL=on  implementation=Fabric  dbl_ovrd=off  block_type=accum
  Constant : xbsIndex_r4/Constant  const=1.0  gui_display_data_type=Boolean  arith_type=Boolean  n_bits=16  bin_pt=14  preci_type=Single  exp_width=8  frac_width=24  explicit_period=on  period=1  equ=P=C  opselect=C  inp2=PCIN>>17  opr=+  inp1=P  carry=CIN  dbl_ovrd=off  block_type=constant
  Delay1 : xbsIndex_r4/Delay  rst=off  infoeditControl=Selection of Reset will increase slice count due to use of real FFs and instead of SRLs  en=off  latency=1  reg_retiming=off  dbl_ovrd=off  block_type=delay
  Delay2 : xbsIndex_r4/Delay  rst=off  infoeditControl=Selection of Reset will increase slice count due to use of real FFs and instead of SRLs  en=off  latency=8  reg_retiming=off  dbl_ovrd=off  block_type=delay
  Mult : xbsIndex_r4/Mult  precision=Full  arith_type="Signed  (2's comp)"  n_bits=16  bin_pt=14  quantization=Truncate  overflow=Wrap  en=off  latency=0  use_behavioral_HDL=off  opt=Speed  use_embedded=on  optimum_pipeline=off  pipeline=on  dbl_ovrd=off  use_rpm=on  placement_style=Triangular  block_type=mult
  Mux : xbsIndex_r4/Mux  inputs=2  en=off  latency=0  precision=Full  arith_type=Unsigned  n_bits=16  bin_pt=14  quantization=Truncate  overflow=Wrap  dbl_ovrd=off  block_type=mux
  B1 : Outport
  C1 : Outport  Port=2
  wires:
  A/1 -> Mult/2
  B/1 -> Delay1/1, Mult/1
  Mult/1 -> Accumulator/1
  Delay1/1 -> B1/1
  reset/1 -> Accumulator/2
  Accumulator/1 -> Mux/2
  Mux/1 -> C1/1
  Constant/1 -> Delay2/1
  Delay2/1 -> Mux/1
  pre_input/1 -> Mux/3

== system ELEC522_PROJECT2/Matrix Multiplication module/PE: MAC21 ==
  B : Inport
  A : Inport  Port=2
  reset : Inport  Port=3
  pre_input : Inport  Port=4
  Accumulator : xbsIndex_r4/Accumulator  operation=Add  n_bits=28  overflow=Wrap  scale=1  rst=on  hasbypass=off  infoeditControl=reset for floating point data type must be asserted for a minimum of 2 cycles  en=off  latency=1  msb_inp=100  msb=100  lsb=-100  use_behavioral_HDL=on  implementation=Fabric  dbl_ovrd=off  block_type=accum
  Constant : xbsIndex_r4/Constant  const=1.0  gui_display_data_type=Boolean  arith_type=Boolean  n_bits=16  bin_pt=14  preci_type=Single  exp_width=8  frac_width=24  explicit_period=on  period=1  equ=P=C  opselect=C  inp2=PCIN>>17  opr=+  inp1=P  carry=CIN  dbl_ovrd=off  block_type=constant
  Delay1 : xbsIndex_r4/Delay  rst=off  infoeditControl=Selection of Reset will increase slice count due to use of real FFs and instead of SRLs  en=off  latency=1  reg_retiming=off  dbl_ovrd=off  block_type=delay
  Delay2 : xbsIndex_r4/Delay  rst=off  infoeditControl=Selection of Reset will increase slice count due to use of real FFs and instead of SRLs  en=off  latency=9  reg_retiming=off  dbl_ovrd=off  block_type=delay
  Mult : xbsIndex_r4/Mult  precision=Full  arith_type="Signed  (2's comp)"  n_bits=16  bin_pt=14  quantization=Truncate  overflow=Wrap  en=off  latency=0  use_behavioral_HDL=off  opt=Speed  use_embedded=on  optimum_pipeline=off  pipeline=on  dbl_ovrd=off  use_rpm=on  placement_style=Triangular  block_type=mult
  Mux : xbsIndex_r4/Mux  inputs=2  en=off  latency=0  precision=Full  arith_type=Unsigned  n_bits=16  bin_pt=14  quantization=Truncate  overflow=Wrap  dbl_ovrd=off  block_type=mux
  B1 : Outport
  C1 : Outport  Port=2
  wires:
  A/1 -> Mult/2
  B/1 -> Delay1/1, Mult/1
  Mult/1 -> Accumulator/1
  Delay1/1 -> B1/1
  reset/1 -> Accumulator/2
  Accumulator/1 -> Mux/2
  Mux/1 -> C1/1
  pre_input/1 -> Mux/3
  Constant/1 -> Delay2/1
  Delay2/1 -> Mux/1

== system ELEC522_PROJECT2/Matrix Multiplication module/PE: MAC22 ==
  B : Inport
  A : Inport  Port=2
  reset : Inport  Port=3
  pre_input : Inport  Port=4
  Accumulator : xbsIndex_r4/Accumulator  operation=Add  n_bits=28  overflow=Wrap  scale=1  rst=on  hasbypass=off  infoeditControl=reset for floating point data type must be asserted for a minimum of 2 cycles  en=off  latency=1  msb_inp=100  msb=100  lsb=-100  use_behavioral_HDL=on  implementation=Fabric  dbl_ovrd=off  block_type=accum
  Constant : xbsIndex_r4/Constant  const=1.0  gui_display_data_type=Boolean  arith_type=Boolean  n_bits=16  bin_pt=14  preci_type=Single  exp_width=8  frac_width=24  explicit_period=on  period=1  equ=P=C  opselect=C  inp2=PCIN>>17  opr=+  inp1=P  carry=CIN  dbl_ovrd=off  block_type=constant
  Delay1 : xbsIndex_r4/Delay  rst=off  infoeditControl=Selection of Reset will increase slice count due to use of real FFs and instead of SRLs  en=off  latency=1  reg_retiming=off  dbl_ovrd=off  block_type=delay
  Delay2 : xbsIndex_r4/Delay  rst=off  infoeditControl=Selection of Reset will increase slice count due to use of real FFs and instead of SRLs  en=off  latency=10  reg_retiming=off  dbl_ovrd=off  block_type=delay
  Mult : xbsIndex_r4/Mult  precision=Full  arith_type="Signed  (2's comp)"  n_bits=16  bin_pt=14  quantization=Truncate  overflow=Wrap  en=off  latency=0  use_behavioral_HDL=off  opt=Speed  use_embedded=on  optimum_pipeline=off  pipeline=on  dbl_ovrd=off  use_rpm=on  placement_style=Triangular  block_type=mult
  Mux : xbsIndex_r4/Mux  inputs=2  en=off  latency=0  precision=Full  arith_type=Unsigned  n_bits=16  bin_pt=14  quantization=Truncate  overflow=Wrap  dbl_ovrd=off  block_type=mux
  B1 : Outport
  C1 : Outport  Port=2
  wires:
  A/1 -> Mult/2
  B/1 -> Delay1/1, Mult/1
  Mult/1 -> Accumulator/1
  Delay1/1 -> B1/1
  reset/1 -> Accumulator/2
  Accumulator/1 -> Mux/2
  Mux/1 -> C1/1
  Constant/1 -> Delay2/1
  Delay2/1 -> Mux/1
  pre_input/1 -> Mux/3

== system ELEC522_PROJECT2/Matrix Multiplication module/PE: MAC23 ==
  B : Inport
  A : Inport  Port=2
  reset : Inport  Port=3
  Accumulator : xbsIndex_r4/Accumulator  operation=Add  n_bits=28  overflow=Wrap  scale=1  rst=on  hasbypass=off  infoeditControl=reset for floating point data type must be asserted for a minimum of 2 cycles  en=off  latency=1  msb_inp=100  msb=100  lsb=-100  use_behavioral_HDL=on  implementation=Fabric  dbl_ovrd=off  block_type=accum
  Mult : xbsIndex_r4/Mult  precision=Full  arith_type="Signed  (2's comp)"  n_bits=16  bin_pt=14  quantization=Truncate  overflow=Wrap  en=off  latency=0  use_behavioral_HDL=off  opt=Speed  use_embedded=on  optimum_pipeline=off  pipeline=on  dbl_ovrd=off  use_rpm=on  placement_style=Triangular  block_type=mult
  C : Outport
  wires:
  A/1 -> Mult/2
  B/1 -> Mult/1
  Mult/1 -> Accumulator/1
  reset/1 -> Accumulator/2
  Accumulator/1 -> C/1

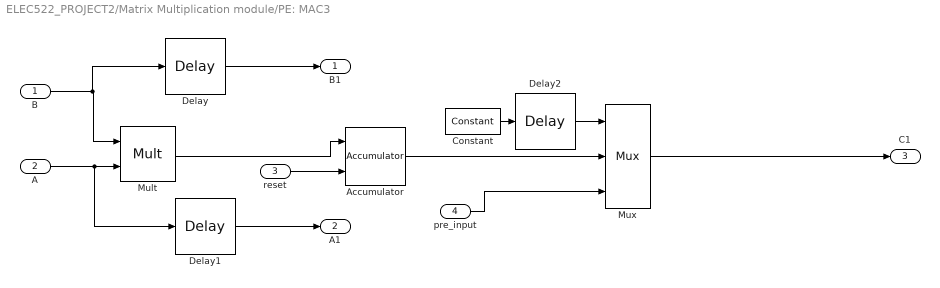
== system ELEC522_PROJECT2/Matrix Multiplication module/PE: MAC3 ==
  B : Inport
  A : Inport  Port=2
  reset : Inport  Port=3
  pre_input : Inport  Port=4
  Accumulator : xbsIndex_r4/Accumulator  operation=Add  n_bits=28  overflow=Wrap  scale=1  rst=on  hasbypass=off  infoeditControl=reset for floating point data type must be asserted for a minimum of 2 cycles  en=off  latency=1  msb_inp=100  msb=100  lsb=-100  use_behavioral_HDL=on  implementation=Fabric  dbl_ovrd=off  block_type=accum
  Constant : xbsIndex_r4/Constant  const=1.0  gui_display_data_type=Boolean  arith_type=Boolean  n_bits=16  bin_pt=14  preci_type=Single  exp_width=8  frac_width=24  explicit_period=on  period=1  equ=P=C  opselect=C  inp2=PCIN>>17  opr=+  inp1=P  carry=CIN  dbl_ovrd=off  block_type=constant
  Delay : xbsIndex_r4/Delay  rst=off  infoeditControl=Selection of Reset will increase slice count due to use of real FFs and instead of SRLs  en=off  latency=1  reg_retiming=off  dbl_ovrd=off  block_type=delay
  Delay1 : xbsIndex_r4/Delay  rst=off  infoeditControl=Selection of Reset will increase slice count due to use of real FFs and instead of SRLs  en=off  latency=1  reg_retiming=off  dbl_ovrd=off  block_type=delay
  Delay2 : xbsIndex_r4/Delay  rst=off  infoeditControl=Selection of Reset will increase slice count due to use of real FFs and instead of SRLs  en=off  latency=8  reg_retiming=off  dbl_ovrd=off  block_type=delay
  Mult : xbsIndex_r4/Mult  precision=Full  arith_type="Signed  (2's comp)"  n_bits=16  bin_pt=14  quantization=Truncate  overflow=Wrap  en=off  latency=0  use_behavioral_HDL=off  opt=Speed  use_embedded=on  optimum_pipeline=off  pipeline=on  dbl_ovrd=off  use_rpm=on  placement_style=Triangular  block_type=mult
  Mux : xbsIndex_r4/Mux  inputs=2  en=off  latency=0  precision=Full  arith_type=Unsigned  n_bits=16  bin_pt=14  quantization=Truncate  overflow=Wrap  dbl_ovrd=off  block_type=mux
  B1 : Outport
  A1 : Outport  Port=2
  C1 : Outport  Port=3
  wires:
  A/1 -> Delay1/1, Mult/2
  B/1 -> Delay/1, Mult/1
  Mult/1 -> Accumulator/1
  Delay1/1 -> A1/1
  Delay/1 -> B1/1
  reset/1 -> Accumulator/2
  Accumulator/1 -> Mux/2
  Constant/1 -> Delay2/1
  Delay2/1 -> Mux/1
  Mux/1 -> C1/1
  pre_input/1 -> Mux/3

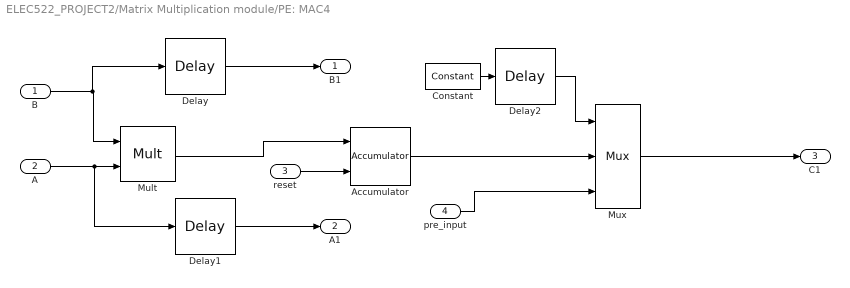
== system ELEC522_PROJECT2/Matrix Multiplication module/PE: MAC4 ==
  B : Inport
  A : Inport  Port=2
  reset : Inport  Port=3
  pre_input : Inport  Port=4
  Accumulator : xbsIndex_r4/Accumulator  operation=Add  n_bits=28  overflow=Wrap  scale=1  rst=on  hasbypass=off  infoeditControl=reset for floating point data type must be asserted for a minimum of 2 cycles  en=off  latency=1  msb_inp=100  msb=100  lsb=-100  use_behavioral_HDL=on  implementation=Fabric  dbl_ovrd=off  block_type=accum
  Constant : xbsIndex_r4/Constant  const=1.0  gui_display_data_type=Boolean  arith_type=Boolean  n_bits=16  bin_pt=14  preci_type=Single  exp_width=8  frac_width=24  explicit_period=on  period=1  equ=P=C  opselect=C  inp2=PCIN>>17  opr=+  inp1=P  carry=CIN  dbl_ovrd=off  block_type=constant
  Delay : xbsIndex_r4/Delay  rst=off  infoeditControl=Selection of Reset will increase slice count due to use of real FFs and instead of SRLs  en=off  latency=1  reg_retiming=off  dbl_ovrd=off  block_type=delay
  Delay1 : xbsIndex_r4/Delay  rst=off  infoeditControl=Selection of Reset will increase slice count due to use of real FFs and instead of SRLs  en=off  latency=1  reg_retiming=off  dbl_ovrd=off  block_type=delay
  Delay2 : xbsIndex_r4/Delay  rst=off  infoeditControl=Selection of Reset will increase slice count due to use of real FFs and instead of SRLs  en=off  latency=6  reg_retiming=off  dbl_ovrd=off  block_type=delay
  Mult : xbsIndex_r4/Mult  precision=Full  arith_type="Signed  (2's comp)"  n_bits=16  bin_pt=14  quantization=Truncate  overflow=Wrap  en=off  latency=0  use_behavioral_HDL=off  opt=Speed  use_embedded=on  optimum_pipeline=off  pipeline=on  dbl_ovrd=off  use_rpm=on  placement_style=Triangular  block_type=mult
  Mux : xbsIndex_r4/Mux  inputs=2  en=off  latency=0  precision=Full  arith_type=Unsigned  n_bits=16  bin_pt=14  quantization=Truncate  overflow=Wrap  dbl_ovrd=off  block_type=mux
  B1 : Outport
  A1 : Outport  Port=2
  C1 : Outport  Port=3
  wires:
  A/1 -> Delay1/1, Mult/2
  B/1 -> Delay/1, Mult/1
  Mult/1 -> Accumulator/1
  Delay1/1 -> A1/1
  Delay/1 -> B1/1
  reset/1 -> Accumulator/2
  Accumulator/1 -> Mux/2
  Mux/1 -> C1/1
  Constant/1 -> Delay2/1
  pre_input/1 -> Mux/3
  Delay2/1 -> Mux/1

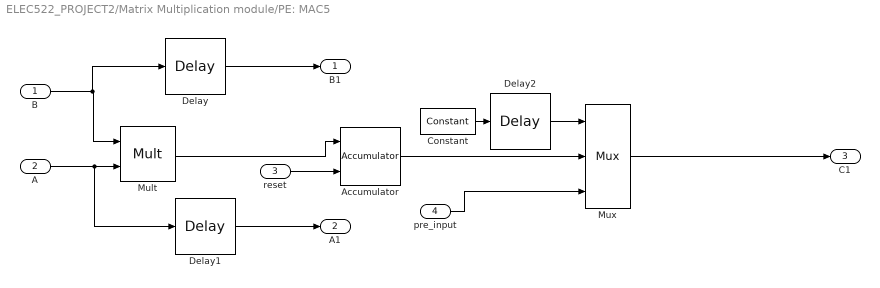
== system ELEC522_PROJECT2/Matrix Multiplication module/PE: MAC5 ==
  B : Inport
  A : Inport  Port=2
  reset : Inport  Port=3
  pre_input : Inport  Port=4
  Accumulator : xbsIndex_r4/Accumulator  operation=Add  n_bits=28  overflow=Wrap  scale=1  rst=on  hasbypass=off  infoeditControl=reset for floating point data type must be asserted for a minimum of 2 cycles  en=off  latency=1  msb_inp=100  msb=100  lsb=-100  use_behavioral_HDL=on  implementation=Fabric  dbl_ovrd=off  block_type=accum
  Constant : xbsIndex_r4/Constant  const=1.0  gui_display_data_type=Boolean  arith_type=Boolean  n_bits=16  bin_pt=14  preci_type=Single  exp_width=8  frac_width=24  explicit_period=on  period=1  equ=P=C  opselect=C  inp2=PCIN>>17  opr=+  inp1=P  carry=CIN  dbl_ovrd=off  block_type=constant
  Delay : xbsIndex_r4/Delay  rst=off  infoeditControl=Selection of Reset will increase slice count due to use of real FFs and instead of SRLs  en=off  latency=1  reg_retiming=off  dbl_ovrd=off  block_type=delay
  Delay1 : xbsIndex_r4/Delay  rst=off  infoeditControl=Selection of Reset will increase slice count due to use of real FFs and instead of SRLs  en=off  latency=1  reg_retiming=off  dbl_ovrd=off  block_type=delay
  Delay2 : xbsIndex_r4/Delay  rst=off  infoeditControl=Selection of Reset will increase slice count due to use of real FFs and instead of SRLs  en=off  latency=7  reg_retiming=off  dbl_ovrd=off  block_type=delay
  Mult : xbsIndex_r4/Mult  precision=Full  arith_type="Signed  (2's comp)"  n_bits=16  bin_pt=14  quantization=Truncate  overflow=Wrap  en=off  latency=0  use_behavioral_HDL=off  opt=Speed  use_embedded=on  optimum_pipeline=off  pipeline=on  dbl_ovrd=off  use_rpm=on  placement_style=Triangular  block_type=mult
  Mux : xbsIndex_r4/Mux  inputs=2  en=off  latency=0  precision=Full  arith_type=Unsigned  n_bits=16  bin_pt=14  quantization=Truncate  overflow=Wrap  dbl_ovrd=off  block_type=mux
  B1 : Outport
  A1 : Outport  Port=2
  C1 : Outport  Port=3
  wires:
  A/1 -> Delay1/1, Mult/2
  B/1 -> Delay/1, Mult/1
  Mult/1 -> Accumulator/1
  Delay1/1 -> A1/1
  Delay/1 -> B1/1
  reset/1 -> Accumulator/2
  Accumulator/1 -> Mux/2
  Mux/1 -> C1/1
  Constant/1 -> Delay2/1
  Delay2/1 -> Mux/1
  pre_input/1 -> Mux/3

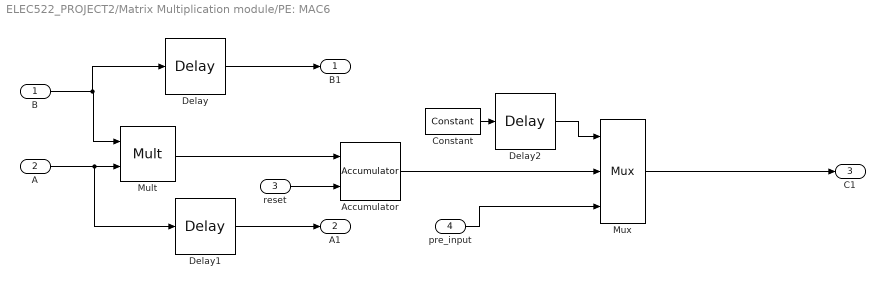
== system ELEC522_PROJECT2/Matrix Multiplication module/PE: MAC6 ==
  B : Inport
  A : Inport  Port=2
  reset : Inport  Port=3
  pre_input : Inport  Port=4
  Accumulator : xbsIndex_r4/Accumulator  operation=Add  n_bits=28  overflow=Wrap  scale=1  rst=on  hasbypass=off  infoeditControl=reset for floating point data type must be asserted for a minimum of 2 cycles  en=off  latency=1  msb_inp=100  msb=100  lsb=-100  use_behavioral_HDL=on  implementation=Fabric  dbl_ovrd=off  block_type=accum
  Constant : xbsIndex_r4/Constant  const=1.0  gui_display_data_type=Boolean  arith_type=Boolean  n_bits=16  bin_pt=14  preci_type=Single  exp_width=8  frac_width=24  explicit_period=on  period=1  equ=P=C  opselect=C  inp2=PCIN>>17  opr=+  inp1=P  carry=CIN  dbl_ovrd=off  block_type=constant
  Delay : xbsIndex_r4/Delay  rst=off  infoeditControl=Selection of Reset will increase slice count due to use of real FFs and instead of SRLs  en=off  latency=1  reg_retiming=off  dbl_ovrd=off  block_type=delay
  Delay1 : xbsIndex_r4/Delay  rst=off  infoeditControl=Selection of Reset will increase slice count due to use of real FFs and instead of SRLs  en=off  latency=1  reg_retiming=off  dbl_ovrd=off  block_type=delay
  Delay2 : xbsIndex_r4/Delay  rst=off  infoeditControl=Selection of Reset will increase slice count due to use of real FFs and instead of SRLs  en=off  latency=7  reg_retiming=off  dbl_ovrd=off  block_type=delay
  Mult : xbsIndex_r4/Mult  precision=Full  arith_type="Signed  (2's comp)"  n_bits=16  bin_pt=14  quantization=Truncate  overflow=Wrap  en=off  latency=0  use_behavioral_HDL=off  opt=Speed  use_embedded=on  optimum_pipeline=off  pipeline=on  dbl_ovrd=off  use_rpm=on  placement_style=Triangular  block_type=mult
  Mux : xbsIndex_r4/Mux  inputs=2  en=off  latency=0  precision=Full  arith_type=Unsigned  n_bits=16  bin_pt=14  quantization=Truncate  overflow=Wrap  dbl_ovrd=off  block_type=mux
  B1 : Outport
  A1 : Outport  Port=2
  C1 : Outport  Port=3
  wires:
  A/1 -> Delay1/1, Mult/2
  B/1 -> Delay/1, Mult/1
  Mult/1 -> Accumulator/1
  Delay1/1 -> A1/1
  Delay/1 -> B1/1
  reset/1 -> Accumulator/2
  Accumulator/1 -> Mux/2
  Mux/1 -> C1/1
  Constant/1 -> Delay2/1
  Delay2/1 -> Mux/1
  pre_input/1 -> Mux/3

== system ELEC522_PROJECT2/Matrix Multiplication module/PE: MAC7 ==
  B : Inport
  A : Inport  Port=2
  reset : Inport  Port=3
  pre_input : Inport  Port=4
  Accumulator : xbsIndex_r4/Accumulator  operation=Add  n_bits=28  overflow=Wrap  scale=1  rst=on  hasbypass=off  infoeditControl=reset for floating point data type must be asserted for a minimum of 2 cycles  en=off  latency=1  msb_inp=100  msb=100  lsb=-100  use_behavioral_HDL=on  implementation=Fabric  dbl_ovrd=off  block_type=accum
  Constant : xbsIndex_r4/Constant  const=1.0  gui_display_data_type=Boolean  arith_type=Boolean  n_bits=16  bin_pt=14  preci_type=Single  exp_width=8  frac_width=24  explicit_period=on  period=1  equ=P=C  opselect=C  inp2=PCIN>>17  opr=+  inp1=P  carry=CIN  dbl_ovrd=off  block_type=constant
  Delay : xbsIndex_r4/Delay  rst=off  infoeditControl=Selection of Reset will increase slice count due to use of real FFs and instead of SRLs  en=off  latency=1  reg_retiming=off  dbl_ovrd=off  block_type=delay
  Delay1 : xbsIndex_r4/Delay  rst=off  infoeditControl=Selection of Reset will increase slice count due to use of real FFs and instead of SRLs  en=off  latency=1  reg_retiming=off  dbl_ovrd=off  block_type=delay
  Delay2 : xbsIndex_r4/Delay  rst=off  infoeditControl=Selection of Reset will increase slice count due to use of real FFs and instead of SRLs  en=off  latency=8  reg_retiming=off  dbl_ovrd=off  block_type=delay
  Mult : xbsIndex_r4/Mult  precision=Full  arith_type="Signed  (2's comp)"  n_bits=16  bin_pt=14  quantization=Truncate  overflow=Wrap  en=off  latency=0  use_behavioral_HDL=off  opt=Speed  use_embedded=on  optimum_pipeline=off  pipeline=on  dbl_ovrd=off  use_rpm=on  placement_style=Triangular  block_type=mult
  Mux : xbsIndex_r4/Mux  inputs=2  en=off  latency=0  precision=Full  arith_type=Unsigned  n_bits=16  bin_pt=14  quantization=Truncate  overflow=Wrap  dbl_ovrd=off  block_type=mux
  B1 : Outport
  A1 : Outport  Port=2
  C1 : Outport  Port=3
  wires:
  A/1 -> Delay1/1, Mult/2
  B/1 -> Delay/1, Mult/1
  Mult/1 -> Accumulator/1
  Delay1/1 -> A1/1
  Delay/1 -> B1/1
  reset/1 -> Accumulator/2
  Accumulator/1 -> Mux/2
  Mux/1 -> C1/1
  Constant/1 -> Delay2/1
  Delay2/1 -> Mux/1
  pre_input/1 -> Mux/3
